simulink model "Comparison_and_analysis"  (R2024a)
settings: Solver=ode23t  StartTime=0.0  StopTime=24  MaxStep=1e-4  RelTol=1e-3
libraries: SignalEditorBlockLib x2, spsGroundLib x2, spsPVArrayLib x2, spsCurrentMeasurementLib x2, spsSeriesRLCBranchLib x2, spsVoltageMeasurementLib x2, sps_lib x1
Description:
  | Comparative analysis on Dual-Axis PV panel vs Fixed PV panel
settings Model: Creator=HP  LastModifiedBy=Asus
settings SolverCC: AlgebraicLoopSolver=TrustRegion
settings DataIOCC: ReturnWorkspaceOutputs=off
settings DebuggingCC: UnconnectedInputMsg=warning  UnconnectedOutputMsg=warning  UnconnectedLineMsg=warning  ArithmeticOperatorsInVariantConditions=warning
settings ModelReferenceCC: EnableRefExpFcnMdlSchedulingChecks=on
settings SFSimCC: SimUseLocalCustomCode=off  CustomCodeUndefinedFunction=UseInterfaceOnly
settings RTWCC: RTWUseLocalCustomCode=off  GPUComputeCapability=3.5
settings CodeAppCC: StateflowObjectComments=on
settings SimscapeCC: SimscapeNormalizeSystem=off

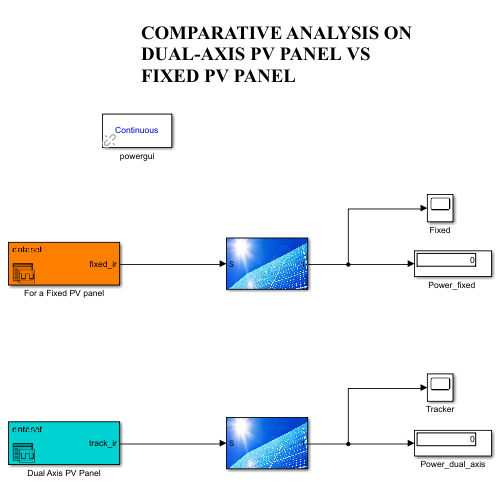
[thumbnail: Simulink's stored preview of the top-level diagram]
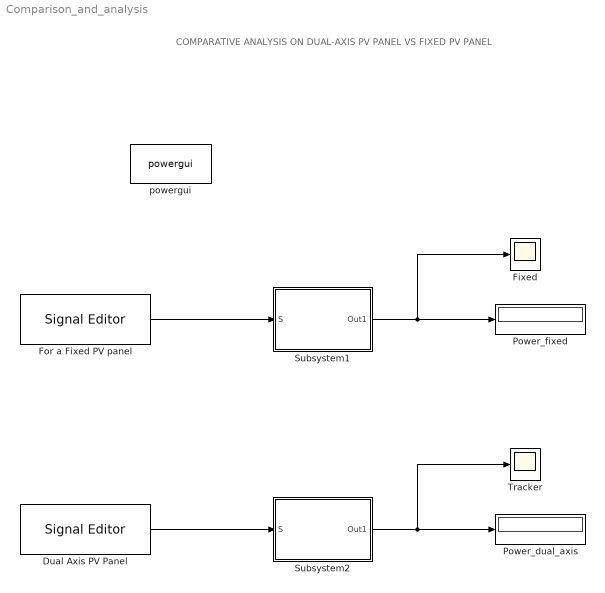
== system Comparison_and_analysis ==
  note: COMPARATIVE ANALYSIS ON DUAL-AXIS PV PANEL VS FIXED PV PANEL
  Dual Axis PV Panel : SignalEditorBlockLib/Signal Editor  FileName=track_ir_data.mat  ActiveScenario=dataset  ActiveSignal=track_ir  IsBus=off  OutputBusObjectStr=Bus: BusObject  SampleTime=0  Interpolate=off  ZeroCross=off  OutputAfterFinalValue=Holding final value  Unit=inherit  PreserveSignalName=on  ApplySigPropsToAllScenarios=on  ApplySigPropsToAllSignals=off
  Fixed : Scope
  For a Fixed PV panel : SignalEditorBlockLib/Signal Editor  FileName=fixed_ir_data.mat  ActiveScenario=dataset  ActiveSignal=fixed_ir  IsBus=off  OutputBusObjectStr=Bus: BusObject  SampleTime=0  Interpolate=off  ZeroCross=off  OutputAfterFinalValue=Setting to zero  Unit=inherit  PreserveSignalName=on  ApplySigPropsToAllScenarios=on  ApplySigPropsToAllSignals=off
  Power_dual_axis : Display
  "Power_fixed " : Display
  Subsystem1 : Subsystem
      mask Display: image('pv_image.jpg');
  Subsystem2 : Subsystem
      mask Display: image('pv_image.jpg');
  Tracker : Scope
  powergui : sps_lib/powergui  Priority=1  SimulationMode=Continuous  SampleTime=50e-6  frequency=60  Iterations=50  frequencyindice=0  Pbase=100e6  ErrMax=1e-4  UnitsV=kV  UnitsW=MW  buscounter=0  FunctionMessages=off  echomessages=off  EnableUseOfTLC=off  CurrentSourceSwitches=off  DisableSnubberDevices=off  DisableRonSwitches=off  DisableVfSwitches=off  DisplayEquations=off  AutomaticDiscreteSolvers=off  SolverType=Tustin/Backward Euler (TBE)  Interpol=off  ExternalGateDelay=off  methode=off  Ts=100  x0status=blocks  SPID=on  SwTol=0  HookPort=off  NonlinearTolerance=1e-4  nMaxIteration=100  ContinueOnMaxIteration=off  RestoreLinks=warning  ResistiveCurrentMeasurement=off  Frange=[0:2:500]  Ylog=off  Xlog=on  ShowGrid=off  save=off  variable=ZData  structure=0  ZoomFFT=off  StartTime=0.0  cycles=1  DisplayStyle=1  fundamental=60  FreqAxis=off  MaxFrequency=1000  frequencyindicesteady=1  RmsSteady=1  display=off
  wires:
  Subsystem1/1(Out1) -> "Power_fixed "/1, Fixed/1
  For a Fixed PV panel/1 -> Subsystem1/1(S)
  Dual Axis PV Panel/1 -> Subsystem2/1(S)
  Subsystem2/1(Out1) -> Power_dual_axis/1, Tracker/1

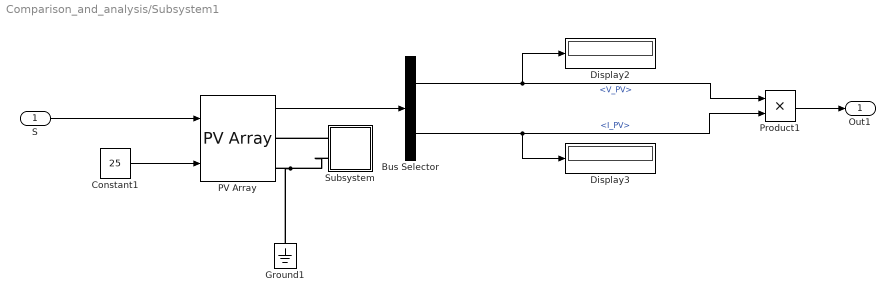
== system Comparison_and_analysis/Subsystem1 ==
  S : Inport
  Bus Selector : BusSelector  OutputSignals=V_PV,I_PV
  Constant1 : Constant  Value=25
  Display2 : Display
  Display3 : Display
  Ground1 : spsGroundLib/Ground  LConnTagsString=a
  PV Array : spsPVArrayLib/PV Array  Npar=1  Nser=1  PlotType=array @ 1000 W/m2 & specified temperatures  S_vec="[ 1000  500  100 ]"  Temp_C_vec="[ 45 25  ]"  ModuleName=User-defined  PlotWhenSelected=off  Pm=200.112  Ncell=54  Voc=32.9  Isc=8.21  Vm=26.4  Im=7.58  beta_Voc_pc=-0.36099  alpha_Isc_pc=0.102  beta_Voc=-0.11877  alpha_Isc=0.0083742  IL=8.2311  I0=3.0465e-10  nI=0.98858  Rsh=126.9934  Rs=0.32653  RobustModel=off  RobustCellTemperature=313.3991  BAL=off  Tc=1e-6  Tfilter=5e-5
  Product1 : Product
  Subsystem : Subsystem
  Out1 : Outport
  wires:
  Bus Selector/2 -> Product1/2, Display3/1  "<I_PV>"
  PV Array/1 -> Bus Selector/1
  Product1/1 -> Out1/1
  Bus Selector/1 -> Product1/1, Display2/1  "<V_PV>"
  Constant1/1 -> PV Array/2
  S/1 -> PV Array/1
  connections:
  Ground1/LConn1 -- Subsystem/LConn2 -- PV Array/RConn2
  Subsystem/LConn1 -- PV Array/RConn1

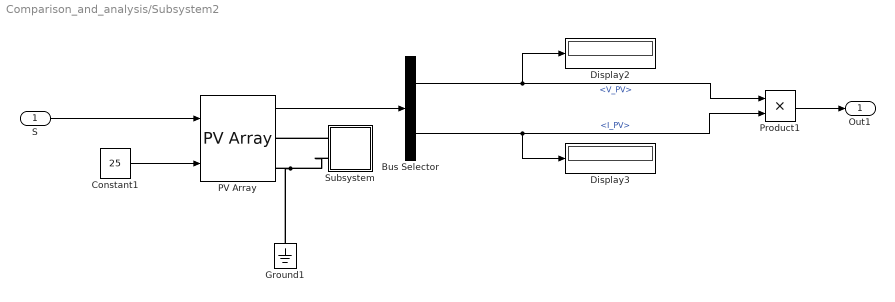
== system Comparison_and_analysis/Subsystem2 ==
  S : Inport
  Bus Selector : BusSelector  OutputSignals=V_PV,I_PV
  Constant1 : Constant  Value=25
  Display2 : Display
  Display3 : Display
  Ground1 : spsGroundLib/Ground  LConnTagsString=a
  PV Array : spsPVArrayLib/PV Array  Npar=1  Nser=1  PlotType=array @ 1000 W/m2 & specified temperatures  S_vec="[ 1000  500  100 ]"  Temp_C_vec="[ 45 25  ]"  ModuleName=User-defined  PlotWhenSelected=off  Pm=200.112  Ncell=54  Voc=32.9  Isc=8.21  Vm=26.4  Im=7.58  beta_Voc_pc=-0.36099  alpha_Isc_pc=0.102  beta_Voc=-0.11877  alpha_Isc=0.0083742  IL=8.2311  I0=3.0465e-10  nI=0.98858  Rsh=126.9934  Rs=0.32653  RobustModel=off  RobustCellTemperature=313.3991  BAL=off  Tc=1e-6  Tfilter=5e-5
  Product1 : Product
  Subsystem : Subsystem
  Out1 : Outport
  wires:
  Bus Selector/2 -> Product1/2, Display3/1  "<I_PV>"
  PV Array/1 -> Bus Selector/1
  Product1/1 -> Out1/1
  Bus Selector/1 -> Product1/1, Display2/1  "<V_PV>"
  Constant1/1 -> PV Array/2
  S/1 -> PV Array/1
  connections:
  Ground1/LConn1 -- PV Array/RConn2 -- Subsystem/LConn2
  Subsystem/LConn1 -- PV Array/RConn1

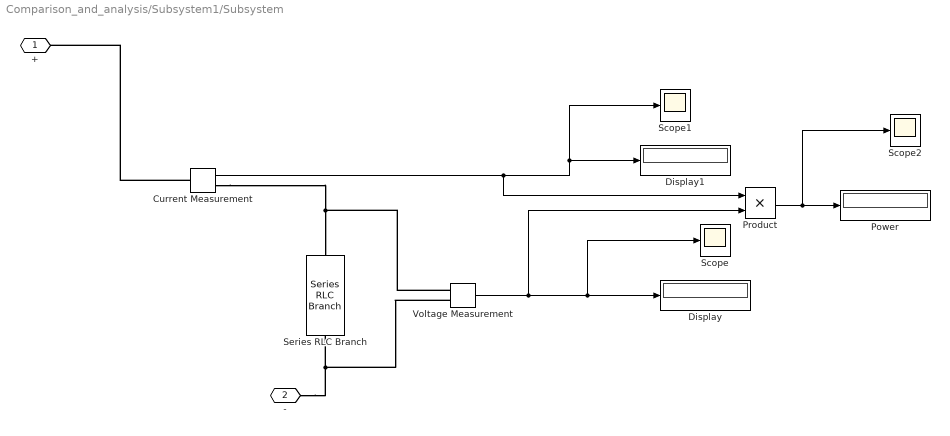
== system Comparison_and_analysis/Subsystem1/Subsystem ==
  Current Measurement : spsCurrentMeasurementLib/Current Measurement  PhasorSimulation=off  OutputType=Complex  PSBequivalent=0
  Display : Display
  Display1 : Display
  Power : Display
  Product : Product
  Scope : Scope
  Scope1 : Scope
  Scope2 : Scope
  Series RLC Branch : spsSeriesRLCBranchLib/Series RLC Branch  LConnTagsString=__new0  RConnTagsString=__new0  BranchType=R  Resistance=3.48  Inductance=1e-3  SetiL0=off  InitialCurrent=0  Capacitance=1e-6  Setx0=off  InitialVoltage=0  Measurements=None
  Voltage Measurement : spsVoltageMeasurementLib/Voltage Measurement  PhasorSimulation=off  OutputType=Complex  PSBequivalent=0
  + : PMIOPort  Side=Left
  - : PMIOPort  Port=2  Side=Left
  wires:
  Current Measurement/1 -> Product/1, Scope1/1, Display1/1
  Voltage Measurement/1 -> Product/2, Scope/1, Display/1
  Product/1 -> Scope2/1, Power/1
  connections:
  Voltage Measurement/LConn2 -- -/RConn1 -- Series RLC Branch/RConn1
  Current Measurement/RConn1 -- Series RLC Branch/LConn1 -- Voltage Measurement/LConn1
  Current Measurement/LConn1 -- +/RConn1

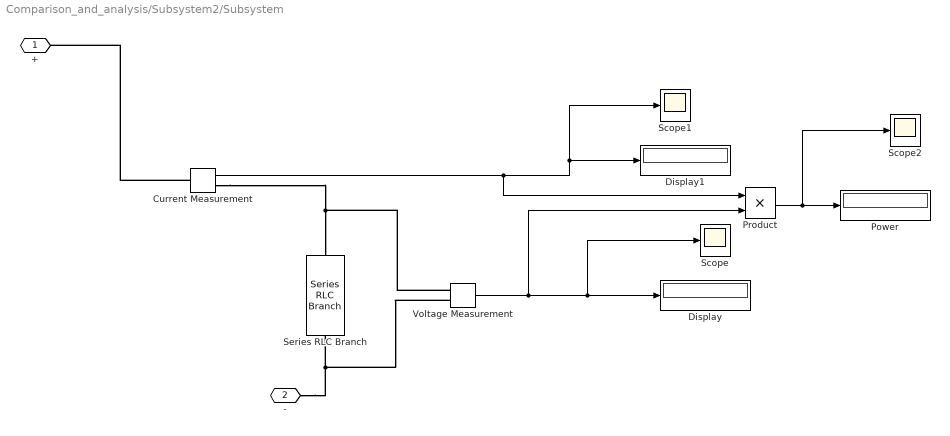
== system Comparison_and_analysis/Subsystem2/Subsystem ==
  Current Measurement : spsCurrentMeasurementLib/Current Measurement  PhasorSimulation=off  OutputType=Complex  PSBequivalent=0
  Display : Display
  Display1 : Display
  Power : Display
  Product : Product
  Scope : Scope
  Scope1 : Scope
  Scope2 : Scope
  Series RLC Branch : spsSeriesRLCBranchLib/Series RLC Branch  LConnTagsString=__new0  RConnTagsString=__new0  BranchType=R  Resistance=3.48  Inductance=1e-3  SetiL0=off  InitialCurrent=0  Capacitance=1e-6  Setx0=off  InitialVoltage=0  Measurements=None
  Voltage Measurement : spsVoltageMeasurementLib/Voltage Measurement  PhasorSimulation=off  OutputType=Complex  PSBequivalent=0
  + : PMIOPort  Side=Left
  - : PMIOPort  Port=2  Side=Left
  wires:
  Current Measurement/1 -> Product/1, Scope1/1, Display1/1
  Voltage Measurement/1 -> Product/2, Scope/1, Display/1
  Product/1 -> Scope2/1, Power/1
  connections:
  Voltage Measurement/LConn2 -- Series RLC Branch/RConn1 -- -/RConn1
  Current Measurement/RConn1 -- Series RLC Branch/LConn1 -- Voltage Measurement/LConn1
  Current Measurement/LConn1 -- +/RConn1
